simulink model "Wheel_Verif"  (R2021b)
settings: Solver=VariableStepAuto  StartTime=0.0  StopTime=10  RelTol=1e-3
values from neighbouring files (symbols this model uses):
  Kt = 14e4    (= 140000)    [CarQuarterParam.m]
  M2 = 20    [CarQuarterParam.m]
settings Model: PacingRate=0.100000  Creator=Reece Bell  LastModifiedBy=reece
settings SolverCC: AlgebraicLoopSolver=TrustRegion
settings DataIOCC: ReturnWorkspaceOutputs=off
settings DebuggingCC: SFMachineParentedDataDiag=warning  ArithmeticOperatorsInVariantConditions=warning
settings SFSimCC: CustomCodeUndefinedFunction=UseInterfaceOnly

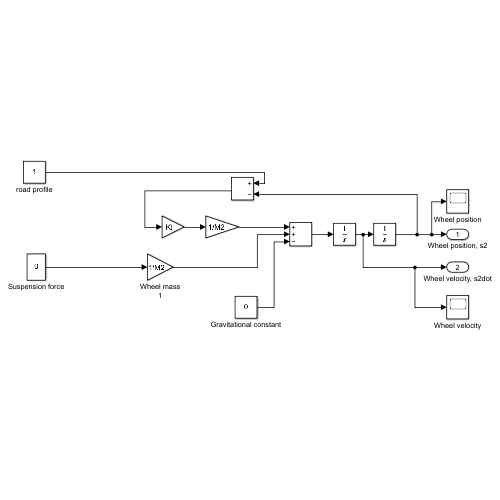
[thumbnail: Simulink's stored preview of the top-level diagram]
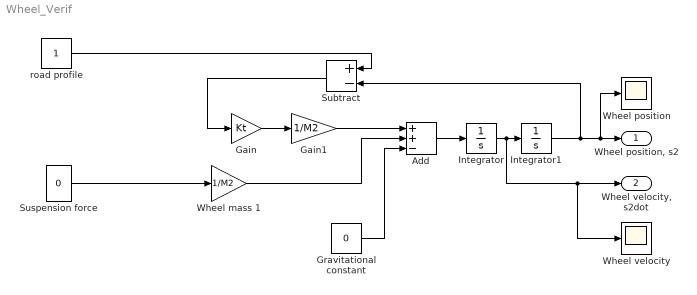
== system Wheel_Verif ==
  Add : Sum  Inputs=++-
  Gain : Gain  Gain=Kt
  Gain1 : Gain  Gain=1/M2
  "Gravitational constant " : Constant  Value=0
  Integrator : Integrator
  Integrator1 : Integrator
  Subtract : Sum  Inputs=+-
  Suspension force : Constant  Value=0
  Wheel mass 1 : Gain  Gain=1/M2
  Wheel position : Scope
  Wheel velocity : Scope
  road profile : Constant
  "Wheel position, s2 " : Outport  VectorParamsAs1DForOutWhenUnconnected=off
  "Wheel velocity, s2dot " : Outport  Port=2  VectorParamsAs1DForOutWhenUnconnected=off
  wires:
  Suspension force/1 -> Wheel mass 1/1
  Integrator/1 -> Wheel velocity/1, "Wheel velocity, s2dot "/1, Integrator1/1
  Wheel mass 1/1 -> Add/2
  "Gravitational constant "/1 -> Add/3
  road profile/1 -> Subtract/1
  Integrator1/1 -> Subtract/2, Wheel position/1, "Wheel position, s2 "/1
  Add/1 -> Integrator/1
  Gain/1 -> Gain1/1
  Subtract/1 -> Gain/1
  Gain1/1 -> Add/1
